simulink model "SAR_ADC_Resistive_DAC_SinInput_HighSpeed_12072024"  (R2022a)
settings: Solver=VariableStepAuto  StartTime=0.0  StopTime=5e-5  RelTol=1e-3
libraries: fl_lib x93, nesl_utility x28, simulink_extras x11, ee_lib x10
settings Model: Creator=subha  LastModifiedBy=subha

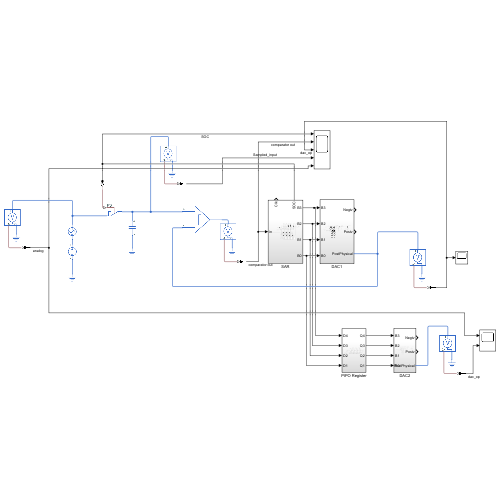
[thumbnail: Simulink's stored preview of the top-level diagram]
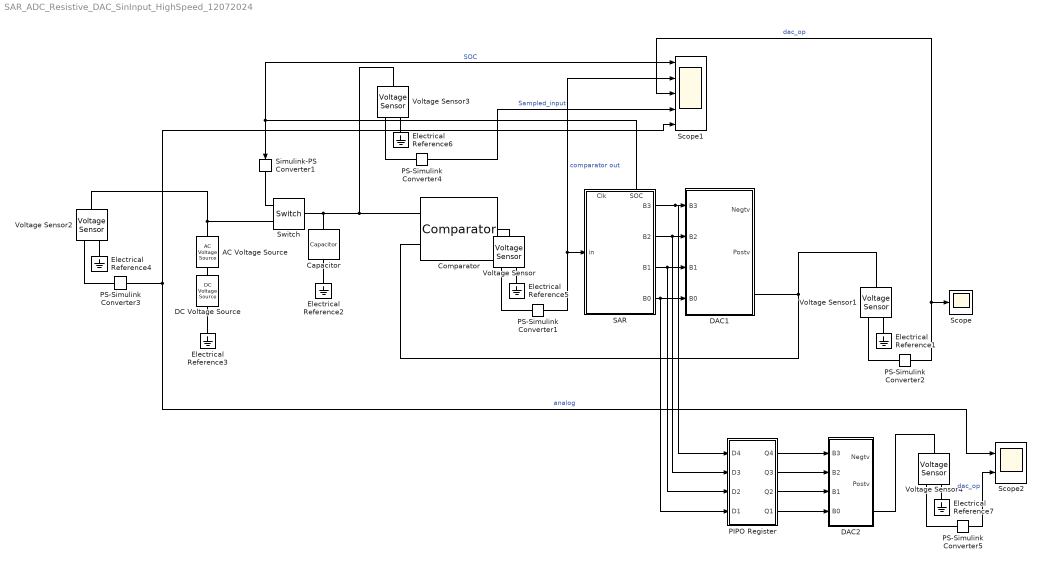
== system SAR_ADC_Resistive_DAC_SinInput_HighSpeed_12072024 ==
  AC Voltage Source : fl_lib/Electrical/Electrical Sources/AC Voltage Source  amp=0.9 V  shift=0 deg  frequency=0.1 MHz  omega=0 rad/s
      settings: SourceProductBaseCode=PW,SS,VE
  Capacitor : fl_lib/Electrical/Electrical Elements/Capacitor  c=1e-9 F  r=1e-6 Ohm  g=0 1/Ohm  i_specify=off  i_priority=None  i=0 A  i_nominal_specify=off  i_nominal_unit=A  i_nominal_value=1  v_specify=off  v_priority=None  v=0 V  v_nominal_specify=off  v_nominal_unit=V  v_nominal_value=1  vc_specify=off  vc_priority=High  vc=0 V  vc_nominal_specify=off  vc_nominal_unit=V  vc_nominal_value=1
      settings: SourceProductBaseCode=PW,SS,VE
  Comparator : ee_lib/Integrated Circuits/Comparator  V_OS=5 mV  C_IN=0 pF  V_OL=0 V  V_OH=5 V  R_OUT=50 Ohm  Delay=0 s
      settings: SourceProductBaseCode=PS  InternalSimscapePortConfiguration="{\"Bottom\":[],\"Left\":[{\"id\":\"p\",\"label\":\"+\",\"type\":\"foundation.electrical.electrical\"},{\"id\":\"n\",\"label\":\"-\",\"type\":\"foundation.electrical.electrical\"}],\"Right\":[{\"id\":\"J\",\"label\":\"\",\"type\":\"foundation.electrical.electrical\"}],\"Top\":[]}"
  DAC1 : Subsystem
  DAC2 : Subsystem
  DC Voltage Source : ee_lib/Additional Components/SPICE Sources/DC Voltage Source  DC=0.9 V
  Electrical Reference{1..7} (7 alike) : fl_lib/Electrical/Electrical Elements/Electrical Reference
      settings: SourceProductBaseCode=PW,SS,VE
  PIPO Register : Subsystem
  PS-Simulink Converter{1..5} (5 alike) : nesl_utility/PS-Simulink Converter  PhysicalDomain=network_engine_domain  SubClassName=ps_output  LeftPortType=input  RightPortType=output  PseudoPeriodic=off  Frequencies=[]  VectorFormat=inherit  Unit=inherit  AffineConversion=off
      settings: SourceProductBaseCode=SS,PW,VE
  SAR : Subsystem
      settings: PortSchema="{\"entries\":[{\"content\":{\"sides\":[{\"content\":{\"connectorIds\":[\"In1\"]},\"type\":\"ConnectorPlacement.EquallySpacedRectSide\",\"uuid\":\"d83d6cbf-1b3c-43c1-b494-336f4d7c2172\"},{\"content\":{\"connectorIds\":[\"Out1\",\"Out2\",\"Out3\",\"Out4\"],\"side\":\"RIGHT\"},\"type\":\"ConnectorPlacement.EquallySpacedRectSide\",\"uuid\":\"5d3d46d0-2210-4ca5-910c-914e08ba7e35\"},{\"content\":{\"connectorIds\":[\"Out5\",\"Out6\"],\"side\":\"TOP\"},\"type\":\"ConnectorPlacement.EquallySpacedRectSide\",\"uuid\":\"cdad274f-a51a-4eb7-9d94-8deabecbb179\"}]},\"type\":\"ConnectorPlacement.EquallySpacedConnector\",\"uuid\":\"7d06527c-7ef1-4315-9939-5225cbeec2df\"}],\"packageUris\":[\"http://schema.mathworks.com/mf0/Connector/R2020b\"],\"version\":\"1.0\"}"
  Scope : Scope
  Scope1 : Scope  NumInputPorts=5
  Scope2 : Scope  NumInputPorts=2
  Simulink-PS Converter1 : nesl_utility/Simulink-PS Converter  PhysicalDomain=network_engine_domain  SubClassName=ps_input  LeftPortType=input  RightPortType=output  PseudoPeriodic=off  Frequencies=[]  NoiseDistribution=none  NoiseParameters=[]  Unit=1  AffineConversion=off  FilteringAndDerivatives=provide  SimscapeFilterOrder=1  InputFilterTimeConstant=0.001  UdotUserProvided=0
      settings: SourceProductBaseCode=SS,PW,VE
  Switch : fl_lib/Electrical/Electrical Elements/Switch  R_closed=0.01 Ohm  G_open=1e-10 1/Ohm  Threshold=0.5  i_specify=off  i_priority=None  i=0 A  i_nominal_specify=off  i_nominal_unit=A  i_nominal_value=1  v_specify=off  v_priority=None  v=0 V  v_nominal_specify=off  v_nominal_unit=V  v_nominal_value=1
      settings: SourceProductBaseCode=PW,SS,VE
  Voltage Sensor{,1..4} (5 alike) : fl_lib/Electrical/Electrical Sensors/Voltage Sensor
      settings: SourceProductBaseCode=PW,SS,VE
  wires:
  PS-Simulink Converter2/1 -> Scope1/3, Scope/1  "dac_op"
  SAR/4(B0) -> DAC1/4(B0), PIPO Register/4(D1)
  PS-Simulink Converter4/1 -> Scope1/4  "Sampled_input"
  PS-Simulink Converter1/1 -> Scope1/2, SAR/1(in)  "comparator out"
  SAR/3(B1) -> PIPO Register/3(D2), DAC1/3(B1)
  SAR/1(B3) -> PIPO Register/1(D4), DAC1/1(B3)
  SAR/2(B2) -> PIPO Register/2(D3), DAC1/2(B2)
  SAR/6(SOC) -> Simulink-PS Converter1/1, Scope1/1  "SOC"
  PS-Simulink Converter3/1 -> Scope2/1, Scope1/5  "analog"
  PIPO Register/1(Q4) -> DAC2/1(B3)
  PIPO Register/2(Q3) -> DAC2/2(B2)
  PIPO Register/3(Q2) -> DAC2/3(B1)
  PIPO Register/4(Q1) -> DAC2/4(B0)
  PS-Simulink Converter5/1 -> Scope2/2  "dac_op"
  connections:
  Capacitor/LConn1 -- Switch/LConn1 -- Comparator/LConn1 -- Voltage Sensor3/LConn1
  Comparator/LConn2 -- DAC1/RConn1 -- Voltage Sensor1/LConn1
  Electrical Reference6/LConn1 -- Voltage Sensor3/RConn2
  Voltage Sensor1/RConn1 -- PS-Simulink Converter2/LConn1
  Simulink-PS Converter1/RConn1 -- Switch/RConn1
  Voltage Sensor3/RConn1 -- PS-Simulink Converter4/LConn1
  Electrical Reference2/LConn1 -- Capacitor/RConn1
  Electrical Reference5/LConn1 -- Voltage Sensor/RConn2
  Voltage Sensor/RConn1 -- PS-Simulink Converter1/LConn1
  Comparator/RConn1 -- Voltage Sensor/LConn1
  Electrical Reference1/LConn1 -- Voltage Sensor1/RConn2
  AC Voltage Source/LConn1 -- Voltage Sensor2/LConn1 -- Switch/RConn2
  DC Voltage Source/LConn1 -- AC Voltage Source/RConn1
  DC Voltage Source/RConn1 -- Electrical Reference3/LConn1
  Electrical Reference4/LConn1 -- Voltage Sensor2/RConn2
  Voltage Sensor2/RConn1 -- PS-Simulink Converter3/LConn1
  Voltage Sensor4/RConn1 -- PS-Simulink Converter5/LConn1
  Electrical Reference7/LConn1 -- Voltage Sensor4/RConn2
  DAC2/RConn1 -- Voltage Sensor4/LConn1

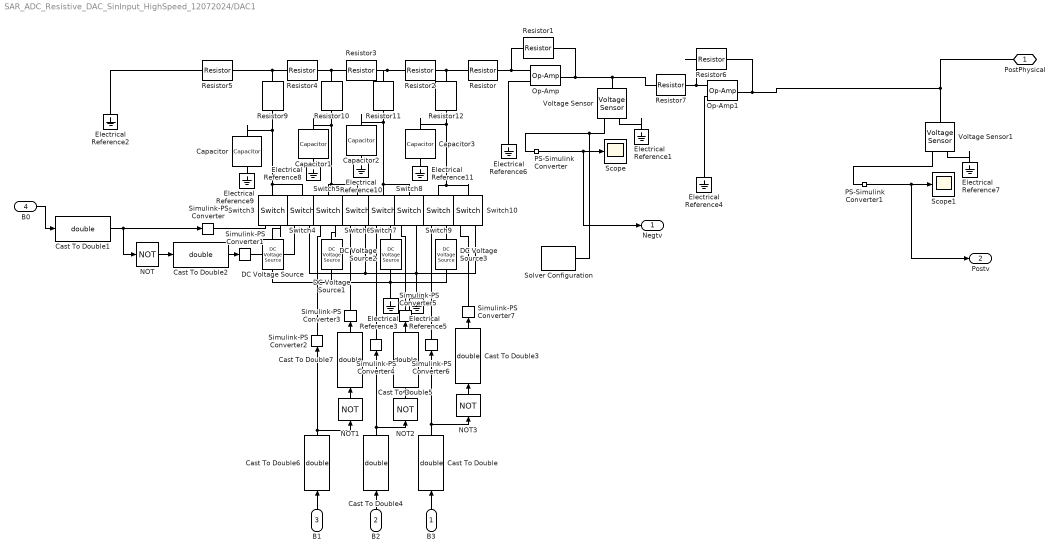
== system SAR_ADC_Resistive_DAC_SinInput_HighSpeed_12072024/DAC1 ==
  B3 : Inport
  B2 : Inport  Port=2
  B1 : Inport  Port=3
  B0 : Inport  Port=4
  Capacitor{,1..3} (4 alike) : fl_lib/Electrical/Electrical Elements/Capacitor  c=1e-9 F  r=1e-6 Ohm  g=0 1/Ohm  i_specify=off  i_priority=None  i=0 A  i_nominal_specify=off  i_nominal_unit=A  i_nominal_value=1  v_specify=off  v_priority=None  v=0 V  v_nominal_specify=off  v_nominal_unit=V  v_nominal_value=1  vc_specify=off  vc_priority=High  vc=0 V  vc_nominal_specify=off  vc_nominal_unit=V  vc_nominal_value=1
      settings: SourceProductBaseCode=PW,SS,VE
  Cast To Double{,1..7} (8 alike) : DataTypeConversion  OutDataTypeStr=double  SaturateOnIntegerOverflow=off  RndMeth=Floor
  DC Voltage Source{,1..3} (4 alike) : ee_lib/Additional Components/SPICE Sources/DC Voltage Source  DC=1.8 V
  Electrical Reference{1..11} (11 alike) : fl_lib/Electrical/Electrical Elements/Electrical Reference
      settings: SourceProductBaseCode=PW,SS,VE
  NOT{,1..3} (4 alike) : Logic  Operator=NOT  IconShape=distinctive  AllPortsSameDT=off  OutDataTypeStr=boolean
  Op-Amp : fl_lib/Electrical/Electrical Elements/Op-Amp  outI_specify=off  outI_priority=None  outI=0 A  outI_nominal_specify=off  outI_nominal_unit=A  outI_nominal_value=1
      settings: SourceProductBaseCode=PW,SS,VE
  Op-Amp1 : fl_lib/Electrical/Electrical Elements/Op-Amp  outI_specify=off  outI_priority=None  outI=0 A  outI_nominal_specify=off  outI_nominal_unit=A  outI_nominal_value=1
      settings: SourceProductBaseCode=PW,SS,VE
  PS-Simulink Converter : nesl_utility/PS-Simulink Converter  PhysicalDomain=network_engine_domain  SubClassName=ps_output  LeftPortType=input  RightPortType=output  PseudoPeriodic=off  Frequencies=[]  VectorFormat=inherit  Unit=inherit  AffineConversion=off
      settings: SourceProductBaseCode=SS,PW,VE
  PS-Simulink Converter1 : nesl_utility/PS-Simulink Converter  PhysicalDomain=network_engine_domain  SubClassName=ps_output  LeftPortType=input  RightPortType=output  PseudoPeriodic=off  Frequencies=[]  VectorFormat=inherit  Unit=inherit  AffineConversion=off
      settings: SourceProductBaseCode=SS,PW,VE
  Resistor{,2..4} (4 alike) : fl_lib/Electrical/Electrical Elements/Resistor  R=1 kOhm  i_specify=off  i_priority=None  i=0 A  i_nominal_specify=off  i_nominal_unit=A  i_nominal_value=1  v_specify=off  v_priority=None  v=0 V  v_nominal_specify=off  v_nominal_unit=V  v_nominal_value=1
      settings: SourceProductBaseCode=PW,SS,VE
  Resistor{1,5,9..12} (6 alike) : fl_lib/Electrical/Electrical Elements/Resistor  R=2 kOhm  i_specify=off  i_priority=None  i=0 A  i_nominal_specify=off  i_nominal_unit=A  i_nominal_value=1  v_specify=off  v_priority=None  v=0 V  v_nominal_specify=off  v_nominal_unit=V  v_nominal_value=1
      settings: SourceProductBaseCode=PW,SS,VE
  Resistor6 : fl_lib/Electrical/Electrical Elements/Resistor  R=10 kOhm  i_specify=off  i_priority=None  i=0 A  i_nominal_specify=off  i_nominal_unit=A  i_nominal_value=1  v_specify=off  v_priority=None  v=0 V  v_nominal_specify=off  v_nominal_unit=V  v_nominal_value=1
      settings: SourceProductBaseCode=PW,SS,VE
  Resistor7 : fl_lib/Electrical/Electrical Elements/Resistor  R=10 kOhm  i_specify=off  i_priority=None  i=0 A  i_nominal_specify=off  i_nominal_unit=A  i_nominal_value=1  v_specify=off  v_priority=None  v=0 V  v_nominal_specify=off  v_nominal_unit=V  v_nominal_value=1
      settings: SourceProductBaseCode=PW,SS,VE
  Scope : Scope
  Scope1 : Scope
  Simulink-PS Converter{,1..7} (8 alike) : nesl_utility/Simulink-PS Converter  PhysicalDomain=network_engine_domain  SubClassName=ps_input  LeftPortType=input  RightPortType=output  PseudoPeriodic=off  Frequencies=[]  NoiseDistribution=none  NoiseParameters=[]  Unit=1  AffineConversion=off  FilteringAndDerivatives=provide  SimscapeFilterOrder=1  InputFilterTimeConstant=0.001  UdotUserProvided=0
      settings: SourceProductBaseCode=SS,PW,VE
  Solver Configuration : nesl_utility/Solver Configuration  PhysicalDomain=network_engine_domain  SubClassName=solver  LeftPortType=input  RightPortType=generic  Tones=[]  Harmonics=[]  SimulateNoise=off  Profile=off  UseLocalSampling=off  EnableSwitchedLinearOptims=on  FrequencyDomain=off  UseCCode=off  RelTol=0.001  AbsTol=0.001  MinStep=1e-09  ToWorkspace=off  RevertToSquareIcSolve=off  NumHomotopyIterations=100  PhasorMode=off  PhasorModeNumHarmonics=1  IndexReductionMethod=DerivativeReplacement  DoDC=off  ResidualTolerance=1e-09  UseLocalSolver=off  LocalSolverChoice=NE_BACKWARD_EULER_ADVANCER  LocalSolverSampleTime=0.001  DoFixedCost=off  MaxNonlinIter=3  MaxModeIter=2  ComputeImpulses=off  ImpulseIterations=2  LinearAlgebra=auto  LinearAlgebraNumThread=0  EquationFormulation=NE_TIME_EF  DelaysMemoryBudget=1024  AutomaticFiltering=on  FilteringTimeConstant=0.001  PartitionStorageMethod=AS_NEEDED  PartitionMemoryBudget=1024  PartitionMethod=ROBUST
      settings: SourceProductBaseCode=SS,PW,VE
  Switch{3..10} (8 alike) : fl_lib/Electrical/Electrical Elements/Switch  R_closed=0.01 Ohm  G_open=1e-8 1/Ohm  Threshold=0.5  i_specify=off  i_priority=None  i=0 A  i_nominal_specify=off  i_nominal_unit=A  i_nominal_value=1  v_specify=off  v_priority=None  v=0 V  v_nominal_specify=off  v_nominal_unit=V  v_nominal_value=1
      settings: SourceProductBaseCode=PW,SS,VE
  Voltage Sensor : fl_lib/Electrical/Electrical Sensors/Voltage Sensor
      settings: SourceProductBaseCode=PW,SS,VE
  Voltage Sensor1 : fl_lib/Electrical/Electrical Sensors/Voltage Sensor
      settings: SourceProductBaseCode=PW,SS,VE
  PostPhysical : PMIOPort  Side=Right
  Negtv : Outport
  Postv : Outport  Port=2
  wires:
  PS-Simulink Converter/1 -> Negtv/1, Scope/1
  Cast To Double/1 -> Simulink-PS Converter6/1, NOT3/1
  B3/1 -> Cast To Double/1
  B0/1 -> Cast To Double1/1
  Cast To Double1/1 -> Simulink-PS Converter/1, NOT/1
  NOT/1 -> Cast To Double2/1
  Cast To Double2/1 -> Simulink-PS Converter1/1
  Cast To Double3/1 -> Simulink-PS Converter7/1
  NOT3/1 -> Cast To Double3/1
  B2/1 -> Cast To Double4/1
  Cast To Double4/1 -> NOT2/1, Simulink-PS Converter4/1
  NOT2/1 -> Cast To Double5/1
  Cast To Double5/1 -> Simulink-PS Converter5/1
  B1/1 -> Cast To Double6/1
  Cast To Double6/1 -> NOT1/1, Simulink-PS Converter2/1
  NOT1/1 -> Cast To Double7/1
  Cast To Double7/1 -> Simulink-PS Converter3/1
  PS-Simulink Converter1/1 -> Postv/1, Scope1/1
  connections:
  Voltage Sensor/RConn1 -- Solver Configuration/RConn1 -- PS-Simulink Converter/LConn1
  DC Voltage Source/RConn1 -- DC Voltage Source1/RConn1 -- DC Voltage Source2/RConn1 -- Electrical Reference3/LConn1 -- DC Voltage Source3/RConn1
  Resistor3/RConn1 -- Resistor2/LConn1 -- Resistor11/LConn1
  Resistor4/RConn1 -- Resistor10/LConn1 -- Resistor3/LConn1
  Resistor5/RConn1 -- Resistor4/LConn1 -- Resistor9/LConn1
  Electrical Reference1/LConn1 -- Voltage Sensor/RConn2
  Resistor2/RConn1 -- Resistor/LConn1 -- Resistor12/LConn1
  Op-Amp/RConn1 -- Resistor7/LConn1 -- Voltage Sensor/LConn1 -- Resistor1/RConn1
  Resistor/RConn1 -- Resistor1/LConn1 -- Op-Amp/LConn2
  Electrical Reference6/LConn1 -- Op-Amp/LConn1
  Switch3/LConn1 -- Switch4/LConn1 -- Capacitor/LConn1 -- Resistor9/RConn1
  Switch3/RConn2 -- DC Voltage Source/LConn1
  Electrical Reference5/LConn1 -- Switch10/RConn2 -- Switch4/RConn2 -- Switch6/RConn2 -- Switch8/RConn2
  Simulink-PS Converter1/RConn1 -- Switch4/RConn1
  Switch5/LConn1 -- Switch6/LConn1 -- Capacitor1/LConn1 -- Resistor10/RConn1
  Switch5/RConn2 -- DC Voltage Source1/LConn1
  Switch7/LConn1 -- Switch8/LConn1 -- Capacitor2/LConn1 -- Resistor11/RConn1
  Switch7/RConn2 -- DC Voltage Source2/LConn1
  Switch10/LConn1 -- Capacitor3/LConn1 -- Resistor12/RConn1 -- Switch9/LConn1
  Switch9/RConn2 -- DC Voltage Source3/LConn1
  Simulink-PS Converter/RConn1 -- Switch3/RConn1
  Simulink-PS Converter3/RConn1 -- Switch6/RConn1
  Simulink-PS Converter2/RConn1 -- Switch5/RConn1
  Switch7/RConn1 -- Simulink-PS Converter4/RConn1
  Switch8/RConn1 -- Simulink-PS Converter5/RConn1
  Switch9/RConn1 -- Simulink-PS Converter6/RConn1
  Switch10/RConn1 -- Simulink-PS Converter7/RConn1
  Electrical Reference4/LConn1 -- Op-Amp1/LConn1
  Resistor7/RConn1 -- Op-Amp1/LConn2 -- Resistor6/LConn1
  Voltage Sensor1/RConn1 -- PS-Simulink Converter1/LConn1
  Resistor6/RConn1 -- Op-Amp1/RConn1 -- PostPhysical/RConn1 -- Voltage Sensor1/LConn1
  Electrical Reference7/LConn1 -- Voltage Sensor1/RConn2
  Electrical Reference2/LConn1 -- Resistor5/LConn1
  Electrical Reference9/LConn1 -- Capacitor/RConn1
  Electrical Reference8/LConn1 -- Capacitor1/RConn1
  Electrical Reference10/LConn1 -- Capacitor2/RConn1
  Electrical Reference11/LConn1 -- Capacitor3/RConn1

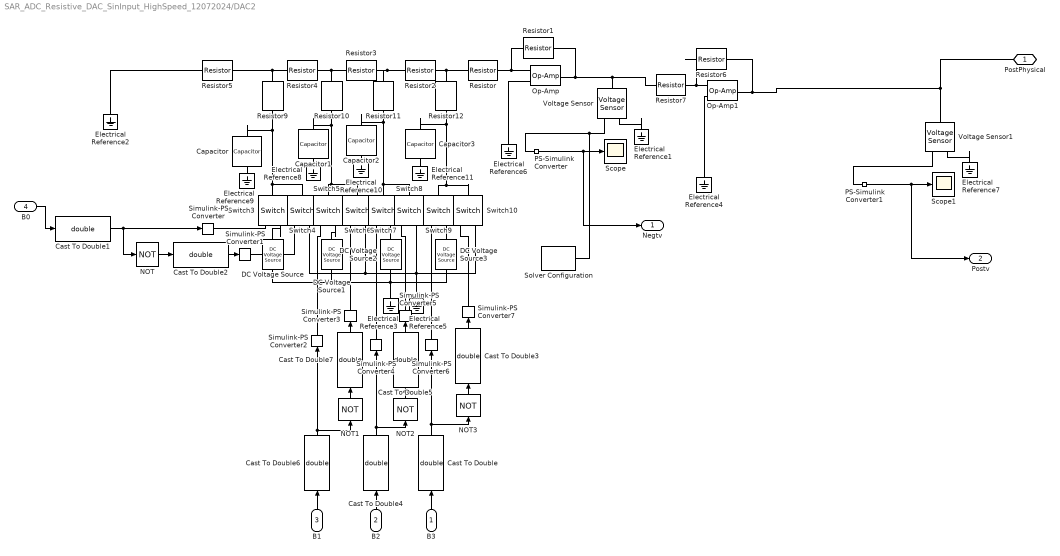
== system SAR_ADC_Resistive_DAC_SinInput_HighSpeed_12072024/DAC2 ==
  B3 : Inport
  B2 : Inport  Port=2
  B1 : Inport  Port=3
  B0 : Inport  Port=4
  Capacitor{,1..3} (4 alike) : fl_lib/Electrical/Electrical Elements/Capacitor  c=1e-9 F  r=1e-6 Ohm  g=0 1/Ohm  i_specify=off  i_priority=None  i=0 A  i_nominal_specify=off  i_nominal_unit=A  i_nominal_value=1  v_specify=off  v_priority=None  v=0 V  v_nominal_specify=off  v_nominal_unit=V  v_nominal_value=1  vc_specify=off  vc_priority=High  vc=0 V  vc_nominal_specify=off  vc_nominal_unit=V  vc_nominal_value=1
      settings: SourceProductBaseCode=PW,SS,VE
  Cast To Double{,1..7} (8 alike) : DataTypeConversion  OutDataTypeStr=double  SaturateOnIntegerOverflow=off  RndMeth=Floor
  DC Voltage Source{,1..3} (4 alike) : ee_lib/Additional Components/SPICE Sources/DC Voltage Source  DC=1.8 V
  Electrical Reference{1..11} (11 alike) : fl_lib/Electrical/Electrical Elements/Electrical Reference
      settings: SourceProductBaseCode=PW,SS,VE
  NOT{,1..3} (4 alike) : Logic  Operator=NOT  IconShape=distinctive  AllPortsSameDT=off  OutDataTypeStr=boolean
  Op-Amp : fl_lib/Electrical/Electrical Elements/Op-Amp  outI_specify=off  outI_priority=None  outI=0 A  outI_nominal_specify=off  outI_nominal_unit=A  outI_nominal_value=1
      settings: SourceProductBaseCode=PW,SS,VE
  Op-Amp1 : fl_lib/Electrical/Electrical Elements/Op-Amp  outI_specify=off  outI_priority=None  outI=0 A  outI_nominal_specify=off  outI_nominal_unit=A  outI_nominal_value=1
      settings: SourceProductBaseCode=PW,SS,VE
  PS-Simulink Converter : nesl_utility/PS-Simulink Converter  PhysicalDomain=network_engine_domain  SubClassName=ps_output  LeftPortType=input  RightPortType=output  PseudoPeriodic=off  Frequencies=[]  VectorFormat=inherit  Unit=inherit  AffineConversion=off
      settings: SourceProductBaseCode=SS,PW,VE
  PS-Simulink Converter1 : nesl_utility/PS-Simulink Converter  PhysicalDomain=network_engine_domain  SubClassName=ps_output  LeftPortType=input  RightPortType=output  PseudoPeriodic=off  Frequencies=[]  VectorFormat=inherit  Unit=inherit  AffineConversion=off
      settings: SourceProductBaseCode=SS,PW,VE
  Resistor{,2..4} (4 alike) : fl_lib/Electrical/Electrical Elements/Resistor  R=1 kOhm  i_specify=off  i_priority=None  i=0 A  i_nominal_specify=off  i_nominal_unit=A  i_nominal_value=1  v_specify=off  v_priority=None  v=0 V  v_nominal_specify=off  v_nominal_unit=V  v_nominal_value=1
      settings: SourceProductBaseCode=PW,SS,VE
  Resistor{1,5,9..12} (6 alike) : fl_lib/Electrical/Electrical Elements/Resistor  R=2 kOhm  i_specify=off  i_priority=None  i=0 A  i_nominal_specify=off  i_nominal_unit=A  i_nominal_value=1  v_specify=off  v_priority=None  v=0 V  v_nominal_specify=off  v_nominal_unit=V  v_nominal_value=1
      settings: SourceProductBaseCode=PW,SS,VE
  Resistor6 : fl_lib/Electrical/Electrical Elements/Resistor  R=10 kOhm  i_specify=off  i_priority=None  i=0 A  i_nominal_specify=off  i_nominal_unit=A  i_nominal_value=1  v_specify=off  v_priority=None  v=0 V  v_nominal_specify=off  v_nominal_unit=V  v_nominal_value=1
      settings: SourceProductBaseCode=PW,SS,VE
  Resistor7 : fl_lib/Electrical/Electrical Elements/Resistor  R=10 kOhm  i_specify=off  i_priority=None  i=0 A  i_nominal_specify=off  i_nominal_unit=A  i_nominal_value=1  v_specify=off  v_priority=None  v=0 V  v_nominal_specify=off  v_nominal_unit=V  v_nominal_value=1
      settings: SourceProductBaseCode=PW,SS,VE
  Scope : Scope
  Scope1 : Scope
  Simulink-PS Converter{,1..7} (8 alike) : nesl_utility/Simulink-PS Converter  PhysicalDomain=network_engine_domain  SubClassName=ps_input  LeftPortType=input  RightPortType=output  PseudoPeriodic=off  Frequencies=[]  NoiseDistribution=none  NoiseParameters=[]  Unit=1  AffineConversion=off  FilteringAndDerivatives=provide  SimscapeFilterOrder=1  InputFilterTimeConstant=0.001  UdotUserProvided=0
      settings: SourceProductBaseCode=SS,PW,VE
  Solver Configuration : nesl_utility/Solver Configuration  PhysicalDomain=network_engine_domain  SubClassName=solver  LeftPortType=input  RightPortType=generic  Tones=[]  Harmonics=[]  SimulateNoise=off  Profile=off  UseLocalSampling=off  EnableSwitchedLinearOptims=on  FrequencyDomain=off  UseCCode=off  RelTol=0.001  AbsTol=0.001  MinStep=1e-09  ToWorkspace=off  RevertToSquareIcSolve=off  NumHomotopyIterations=100  PhasorMode=off  PhasorModeNumHarmonics=1  IndexReductionMethod=DerivativeReplacement  DoDC=off  ResidualTolerance=1e-09  UseLocalSolver=off  LocalSolverChoice=NE_BACKWARD_EULER_ADVANCER  LocalSolverSampleTime=0.001  DoFixedCost=off  MaxNonlinIter=3  MaxModeIter=2  ComputeImpulses=off  ImpulseIterations=2  LinearAlgebra=auto  LinearAlgebraNumThread=0  EquationFormulation=NE_TIME_EF  DelaysMemoryBudget=1024  AutomaticFiltering=on  FilteringTimeConstant=0.001  PartitionStorageMethod=AS_NEEDED  PartitionMemoryBudget=1024  PartitionMethod=ROBUST
      settings: SourceProductBaseCode=SS,PW,VE
  Switch{3..10} (8 alike) : fl_lib/Electrical/Electrical Elements/Switch  R_closed=0.01 Ohm  G_open=1e-8 1/Ohm  Threshold=0.5  i_specify=off  i_priority=None  i=0 A  i_nominal_specify=off  i_nominal_unit=A  i_nominal_value=1  v_specify=off  v_priority=None  v=0 V  v_nominal_specify=off  v_nominal_unit=V  v_nominal_value=1
      settings: SourceProductBaseCode=PW,SS,VE
  Voltage Sensor : fl_lib/Electrical/Electrical Sensors/Voltage Sensor
      settings: SourceProductBaseCode=PW,SS,VE
  Voltage Sensor1 : fl_lib/Electrical/Electrical Sensors/Voltage Sensor
      settings: SourceProductBaseCode=PW,SS,VE
  PostPhysical : PMIOPort  Side=Right
  Negtv : Outport
  Postv : Outport  Port=2
  wires:
  PS-Simulink Converter/1 -> Negtv/1, Scope/1
  Cast To Double/1 -> Simulink-PS Converter6/1, NOT3/1
  B3/1 -> Cast To Double/1
  B0/1 -> Cast To Double1/1
  Cast To Double1/1 -> Simulink-PS Converter/1, NOT/1
  NOT/1 -> Cast To Double2/1
  Cast To Double2/1 -> Simulink-PS Converter1/1
  Cast To Double3/1 -> Simulink-PS Converter7/1
  NOT3/1 -> Cast To Double3/1
  B2/1 -> Cast To Double4/1
  Cast To Double4/1 -> NOT2/1, Simulink-PS Converter4/1
  NOT2/1 -> Cast To Double5/1
  Cast To Double5/1 -> Simulink-PS Converter5/1
  B1/1 -> Cast To Double6/1
  Cast To Double6/1 -> NOT1/1, Simulink-PS Converter2/1
  NOT1/1 -> Cast To Double7/1
  Cast To Double7/1 -> Simulink-PS Converter3/1
  PS-Simulink Converter1/1 -> Postv/1, Scope1/1
  connections:
  Voltage Sensor/RConn1 -- Solver Configuration/RConn1 -- PS-Simulink Converter/LConn1
  DC Voltage Source/RConn1 -- DC Voltage Source1/RConn1 -- DC Voltage Source2/RConn1 -- Electrical Reference3/LConn1 -- DC Voltage Source3/RConn1
  Resistor3/RConn1 -- Resistor2/LConn1 -- Resistor11/LConn1
  Resistor4/RConn1 -- Resistor10/LConn1 -- Resistor3/LConn1
  Resistor5/RConn1 -- Resistor4/LConn1 -- Resistor9/LConn1
  Electrical Reference1/LConn1 -- Voltage Sensor/RConn2
  Resistor2/RConn1 -- Resistor/LConn1 -- Resistor12/LConn1
  Op-Amp/RConn1 -- Resistor7/LConn1 -- Voltage Sensor/LConn1 -- Resistor1/RConn1
  Resistor/RConn1 -- Resistor1/LConn1 -- Op-Amp/LConn2
  Electrical Reference6/LConn1 -- Op-Amp/LConn1
  Switch3/LConn1 -- Switch4/LConn1 -- Capacitor/LConn1 -- Resistor9/RConn1
  Switch3/RConn2 -- DC Voltage Source/LConn1
  Electrical Reference5/LConn1 -- Switch10/RConn2 -- Switch4/RConn2 -- Switch6/RConn2 -- Switch8/RConn2
  Simulink-PS Converter1/RConn1 -- Switch4/RConn1
  Switch5/LConn1 -- Switch6/LConn1 -- Capacitor1/LConn1 -- Resistor10/RConn1
  Switch5/RConn2 -- DC Voltage Source1/LConn1
  Switch7/LConn1 -- Switch8/LConn1 -- Capacitor2/LConn1 -- Resistor11/RConn1
  Switch7/RConn2 -- DC Voltage Source2/LConn1
  Switch10/LConn1 -- Capacitor3/LConn1 -- Resistor12/RConn1 -- Switch9/LConn1
  Switch9/RConn2 -- DC Voltage Source3/LConn1
  Simulink-PS Converter/RConn1 -- Switch3/RConn1
  Simulink-PS Converter3/RConn1 -- Switch6/RConn1
  Simulink-PS Converter2/RConn1 -- Switch5/RConn1
  Switch7/RConn1 -- Simulink-PS Converter4/RConn1
  Switch8/RConn1 -- Simulink-PS Converter5/RConn1
  Switch9/RConn1 -- Simulink-PS Converter6/RConn1
  Switch10/RConn1 -- Simulink-PS Converter7/RConn1
  Electrical Reference4/LConn1 -- Op-Amp1/LConn1
  Resistor7/RConn1 -- Op-Amp1/LConn2 -- Resistor6/LConn1
  Voltage Sensor1/RConn1 -- PS-Simulink Converter1/LConn1
  Resistor6/RConn1 -- Op-Amp1/RConn1 -- PostPhysical/RConn1 -- Voltage Sensor1/LConn1
  Electrical Reference7/LConn1 -- Voltage Sensor1/RConn2
  Electrical Reference2/LConn1 -- Resistor5/LConn1
  Electrical Reference9/LConn1 -- Capacitor/RConn1
  Electrical Reference8/LConn1 -- Capacitor1/RConn1
  Electrical Reference10/LConn1 -- Capacitor2/RConn1
  Electrical Reference11/LConn1 -- Capacitor3/RConn1

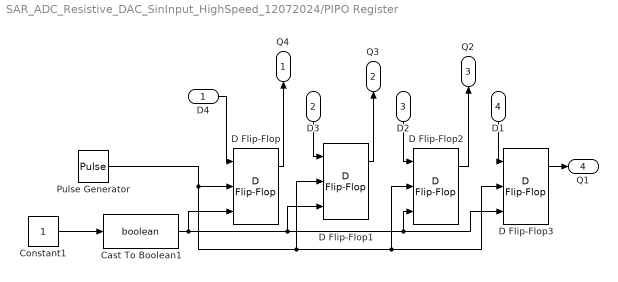
== system SAR_ADC_Resistive_DAC_SinInput_HighSpeed_12072024/PIPO Register ==
  D4 : Inport
  D3 : Inport  Port=2
  D2 : Inport  Port=3
  D1 : Inport  Port=4
  Cast To Boolean1 : DataTypeConversion  OutDataTypeStr=boolean  SaturateOnIntegerOverflow=off  RndMeth=Floor
  Constant1 : Constant
  D Flip-Flop{,1..3} (4 alike) : simulink_extras/Flip Flops/D Flip-Flop
  Pulse Generator : DiscretePulseGenerator  PulseType=Time based  Period=12e-8  PulseWidth=8.3  PhaseDelay=11e-8
  Q4 : Outport
  Q3 : Outport  Port=2
  Q2 : Outport  Port=3
  Q1 : Outport  Port=4
  wires:
  Constant1/1 -> Cast To Boolean1/1
  Pulse Generator/1 -> D Flip-Flop3/2, D Flip-Flop2/2, D Flip-Flop1/2, D Flip-Flop/2
  D1/1 -> D Flip-Flop3/1
  Cast To Boolean1/1 -> D Flip-Flop2/3, D Flip-Flop3/3, D Flip-Flop1/3, D Flip-Flop/3
  D Flip-Flop/1 -> Q4/1
  D Flip-Flop2/1 -> Q2/1
  D2/1 -> D Flip-Flop2/1
  D3/1 -> D Flip-Flop1/1
  D Flip-Flop3/1 -> Q1/1
  D Flip-Flop1/1 -> Q3/1
  D4/1 -> D Flip-Flop/1

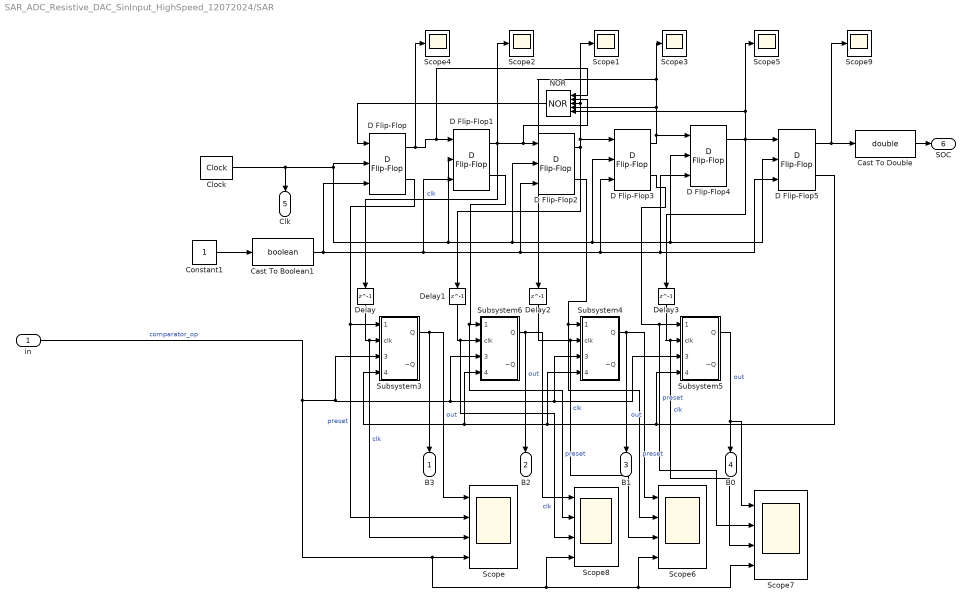
== system SAR_ADC_Resistive_DAC_SinInput_HighSpeed_12072024/SAR ==
  in : Inport
  Cast To Boolean1 : DataTypeConversion  OutDataTypeStr=boolean  SaturateOnIntegerOverflow=off  RndMeth=Floor
  Cast To Double : DataTypeConversion  OutDataTypeStr=double  SaturateOnIntegerOverflow=off  RndMeth=Floor
  Clock : simulink_extras/Flip Flops/Clock  period=2e-8
  Constant1 : Constant
  D Flip-Flop{,1..5} (6 alike) : simulink_extras/Flip Flops/D Flip-Flop
  Delay{,1..3} (4 alike) : Delay  DelayLength=1
  NOR : Logic  Operator=NOR  Inputs=5  IconShape=distinctive  AllPortsSameDT=off  OutDataTypeStr=boolean
  Scope{,6..8} (4 alike) : Scope  NumInputPorts=4
  Scope{1..5,9} (6 alike) : Scope
  Subsystem3 : Subsystem
  Subsystem4 : Subsystem
  Subsystem5 : Subsystem
  Subsystem6 : Subsystem
  B3 : Outport
  B2 : Outport  Port=2
  B1 : Outport  Port=3
  B0 : Outport  Port=4
  Clk : Outport  Port=5
  SOC : Outport  Port=6
  wires:
  D Flip-Flop3/1 -> NOR/4, Delay2/1, Scope3/1, D Flip-Flop4/1
  Clock/1 -> Clk/1, D Flip-Flop/2, D Flip-Flop1/2, D Flip-Flop2/2, D Flip-Flop5/2, D Flip-Flop4/2, D Flip-Flop3/2
  D Flip-Flop3/2 -> Scope7/2, Subsystem5/1(preset)  "preset"
  in/1 -> Scope7/4, Scope6/4, Scope8/4, Scope/4, Subsystem3/3(input), Subsystem6/3(input), Subsystem5/3(input), Subsystem4/3(input)  "comparator_op"
  NOR/1 -> D Flip-Flop/1
  Delay2/1 -> Scope6/3, Subsystem4/2(clk)  "clk"
  Delay3/1 -> Scope7/3, Subsystem5/2(clk)  "clk"
  D Flip-Flop4/1 -> D Flip-Flop5/1, Delay3/1, NOR/5, Scope5/1
  Cast To Boolean1/1 -> D Flip-Flop/3, D Flip-Flop5/3, D Flip-Flop4/3, D Flip-Flop3/3, D Flip-Flop2/3, D Flip-Flop1/3
  D Flip-Flop2/2 -> Scope6/2, Subsystem4/1(preset)  "preset"
  D Flip-Flop1/2 -> Scope8/2, Subsystem6/1(preset)  "preset"
  D Flip-Flop2/1 -> Delay1/1, D Flip-Flop3/1, NOR/3, Scope1/1
  D Flip-Flop1/1 -> Delay/1, NOR/2, D Flip-Flop2/1, Scope2/1  "clk"
  Subsystem6/1(Q) -> B2/1, Scope8/1  "out"
  D Flip-Flop/1 -> Scope4/1, NOR/1, D Flip-Flop1/1
  D Flip-Flop/2 -> Subsystem3/1(preset), Scope/2  "preset"
  Constant1/1 -> Cast To Boolean1/1
  Subsystem4/1(Q) -> B1/1, Scope6/1  "out"
  Subsystem3/1(Q) -> B3/1, Scope/1  "out"
  Delay1/1 -> Scope8/3, Subsystem6/2(clk)  "clk"
  Delay/1 -> Scope/3, Subsystem3/2(clk)  "clk"
  Subsystem5/1(Q) -> B0/1, Scope7/1  "out"
  D Flip-Flop5/2 -> Subsystem3/4(clear), Subsystem6/4(clear), Subsystem4/4(clear), Subsystem5/4(clear)
  D Flip-Flop5/1 -> Cast To Double/1, Scope9/1
  Cast To Double/1 -> SOC/1

== system SAR_ADC_Resistive_DAC_SinInput_HighSpeed_12072024/SAR/Subsystem3 ==
  preset : Inport
  clk : Inport  Port=2
  input : Inport  Port=3
  clear : Inport  Port=4
  NOT : Logic  Operator=NOT  IconShape=distinctive  AllPortsSameDT=off  OutDataTypeStr=boolean
  Subsystem : Subsystem
  Subsystem1 : Subsystem
  Q : Outport
  ~Q : Outport  Port=2
  wires:
  clk/1 -> Subsystem1/3(clock), NOT/1
  Subsystem/1(Q) -> Subsystem1/2(D)
  NOT/1 -> Subsystem/3(clock)
  preset/1 -> Subsystem1/1(preset), Subsystem/1(preset)
  clear/1 -> Subsystem/4(clear), Subsystem1/4(clear)
  input/1 -> Subsystem/2(D)
  Subsystem1/1(Q) -> Q/1  "output"
  Subsystem1/2(~Q) -> ~Q/1

== system SAR_ADC_Resistive_DAC_SinInput_HighSpeed_12072024/SAR/Subsystem4 ==
  preset : Inport
  clk : Inport  Port=2
  input : Inport  Port=3
  clear : Inport  Port=4
  NOT : Logic  Operator=NOT  IconShape=distinctive  AllPortsSameDT=off  OutDataTypeStr=boolean
  Subsystem : Subsystem
  Subsystem1 : Subsystem
  Q : Outport
  ~Q : Outport  Port=2
  wires:
  clk/1 -> Subsystem1/3(clock), NOT/1
  Subsystem/1(Q) -> Subsystem1/2(D)
  NOT/1 -> Subsystem/3(clock)
  preset/1 -> Subsystem1/1(preset), Subsystem/1(preset)
  clear/1 -> Subsystem/4(clear), Subsystem1/4(clear)
  input/1 -> Subsystem/2(D)
  Subsystem1/1(Q) -> Q/1  "output"
  Subsystem1/2(~Q) -> ~Q/1

== system SAR_ADC_Resistive_DAC_SinInput_HighSpeed_12072024/SAR/Subsystem5 ==
  preset : Inport
  clk : Inport  Port=2
  input : Inport  Port=3
  clear : Inport  Port=4
  NOT : Logic  Operator=NOT  IconShape=distinctive  AllPortsSameDT=off  OutDataTypeStr=boolean
  Subsystem : Subsystem
  Subsystem1 : Subsystem
  Q : Outport
  ~Q : Outport  Port=2
  wires:
  clk/1 -> Subsystem1/3(clock), NOT/1
  Subsystem/1(Q) -> Subsystem1/2(D)
  NOT/1 -> Subsystem/3(clock)
  preset/1 -> Subsystem1/1(preset), Subsystem/1(preset)
  clear/1 -> Subsystem/4(clear), Subsystem1/4(clear)
  input/1 -> Subsystem/2(D)
  Subsystem1/1(Q) -> Q/1  "output"
  Subsystem1/2(~Q) -> ~Q/1

== system SAR_ADC_Resistive_DAC_SinInput_HighSpeed_12072024/SAR/Subsystem6 ==
  preset : Inport
  clk : Inport  Port=2
  input : Inport  Port=3
  clear : Inport  Port=4
  NOT : Logic  Operator=NOT  IconShape=distinctive  AllPortsSameDT=off  OutDataTypeStr=boolean
  Subsystem : Subsystem
  Subsystem1 : Subsystem
  Q : Outport
  ~Q : Outport  Port=2
  wires:
  clk/1 -> Subsystem1/3(clock), NOT/1
  Subsystem/1(Q) -> Subsystem1/2(D)
  NOT/1 -> Subsystem/3(clock)
  preset/1 -> Subsystem1/1(preset), Subsystem/1(preset)
  clear/1 -> Subsystem/4(clear), Subsystem1/4(clear)
  input/1 -> Subsystem/2(D)
  Subsystem1/1(Q) -> Q/1  "output"
  Subsystem1/2(~Q) -> ~Q/1

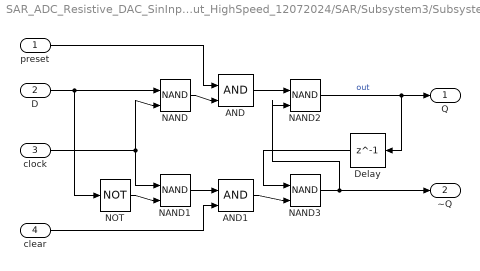
== system SAR_ADC_Resistive_DAC_SinInput_HighSpeed_12072024/SAR/Subsystem3/Subsystem ==
  preset : Inport
  D : Inport  Port=2
  clock : Inport  Port=3
  clear : Inport  Port=4
  AND : Logic  IconShape=distinctive  AllPortsSameDT=off  OutDataTypeStr=boolean
  AND1 : Logic  IconShape=distinctive  AllPortsSameDT=off  OutDataTypeStr=boolean
  Delay : Delay  DelayLength=1
  NAND{,1..3} (4 alike) : Logic  Operator=NAND  IconShape=distinctive  AllPortsSameDT=off  OutDataTypeStr=boolean
  NOT : Logic  Operator=NOT  IconShape=distinctive  AllPortsSameDT=off  OutDataTypeStr=boolean
  Q : Outport
  ~Q : Outport  Port=2
  wires:
  Delay/1 -> NAND3/1
  NOT/1 -> NAND1/2
  NAND1/1 -> AND1/1
  AND/1 -> NAND2/1
  NAND3/1 -> ~Q/1, NAND2/2
  D/1 -> NOT/1, NAND/1
  AND1/1 -> NAND3/2
  NAND/1 -> AND/2
  NAND2/1 -> Q/1, Delay/1  "out"
  clock/1 -> NAND/2, NAND1/1
  preset/1 -> AND/1
  clear/1 -> AND1/2

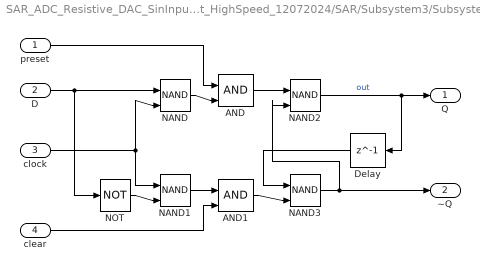
== system SAR_ADC_Resistive_DAC_SinInput_HighSpeed_12072024/SAR/Subsystem3/Subsystem1 ==
  preset : Inport
  D : Inport  Port=2
  clock : Inport  Port=3
  clear : Inport  Port=4
  AND : Logic  IconShape=distinctive  AllPortsSameDT=off  OutDataTypeStr=boolean
  AND1 : Logic  IconShape=distinctive  AllPortsSameDT=off  OutDataTypeStr=boolean
  Delay : Delay  DelayLength=1
  NAND{,1..3} (4 alike) : Logic  Operator=NAND  IconShape=distinctive  AllPortsSameDT=off  OutDataTypeStr=boolean
  NOT : Logic  Operator=NOT  IconShape=distinctive  AllPortsSameDT=off  OutDataTypeStr=boolean
  Q : Outport
  ~Q : Outport  Port=2
  wires:
  Delay/1 -> NAND3/1
  NOT/1 -> NAND1/2
  NAND1/1 -> AND1/1
  AND/1 -> NAND2/1
  NAND3/1 -> ~Q/1, NAND2/2
  D/1 -> NOT/1, NAND/1
  AND1/1 -> NAND3/2
  NAND/1 -> AND/2
  NAND2/1 -> Q/1, Delay/1  "out"
  clock/1 -> NAND/2, NAND1/1
  preset/1 -> AND/1
  clear/1 -> AND1/2

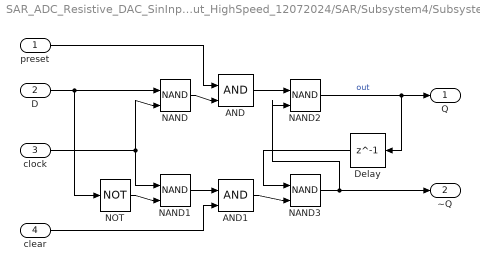
== system SAR_ADC_Resistive_DAC_SinInput_HighSpeed_12072024/SAR/Subsystem4/Subsystem ==
  preset : Inport
  D : Inport  Port=2
  clock : Inport  Port=3
  clear : Inport  Port=4
  AND : Logic  IconShape=distinctive  AllPortsSameDT=off  OutDataTypeStr=boolean
  AND1 : Logic  IconShape=distinctive  AllPortsSameDT=off  OutDataTypeStr=boolean
  Delay : Delay  DelayLength=1
  NAND{,1..3} (4 alike) : Logic  Operator=NAND  IconShape=distinctive  AllPortsSameDT=off  OutDataTypeStr=boolean
  NOT : Logic  Operator=NOT  IconShape=distinctive  AllPortsSameDT=off  OutDataTypeStr=boolean
  Q : Outport
  ~Q : Outport  Port=2
  wires:
  Delay/1 -> NAND3/1
  NOT/1 -> NAND1/2
  NAND1/1 -> AND1/1
  AND/1 -> NAND2/1
  NAND3/1 -> ~Q/1, NAND2/2
  D/1 -> NOT/1, NAND/1
  AND1/1 -> NAND3/2
  NAND/1 -> AND/2
  NAND2/1 -> Q/1, Delay/1  "out"
  clock/1 -> NAND/2, NAND1/1
  preset/1 -> AND/1
  clear/1 -> AND1/2

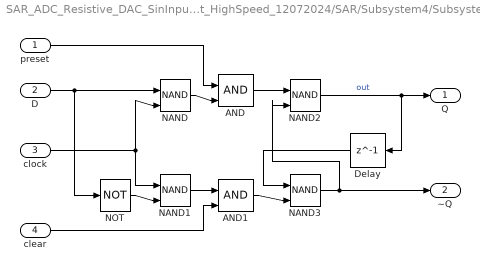
== system SAR_ADC_Resistive_DAC_SinInput_HighSpeed_12072024/SAR/Subsystem4/Subsystem1 ==
  preset : Inport
  D : Inport  Port=2
  clock : Inport  Port=3
  clear : Inport  Port=4
  AND : Logic  IconShape=distinctive  AllPortsSameDT=off  OutDataTypeStr=boolean
  AND1 : Logic  IconShape=distinctive  AllPortsSameDT=off  OutDataTypeStr=boolean
  Delay : Delay  DelayLength=1
  NAND{,1..3} (4 alike) : Logic  Operator=NAND  IconShape=distinctive  AllPortsSameDT=off  OutDataTypeStr=boolean
  NOT : Logic  Operator=NOT  IconShape=distinctive  AllPortsSameDT=off  OutDataTypeStr=boolean
  Q : Outport
  ~Q : Outport  Port=2
  wires:
  Delay/1 -> NAND3/1
  NOT/1 -> NAND1/2
  NAND1/1 -> AND1/1
  AND/1 -> NAND2/1
  NAND3/1 -> ~Q/1, NAND2/2
  D/1 -> NOT/1, NAND/1
  AND1/1 -> NAND3/2
  NAND/1 -> AND/2
  NAND2/1 -> Q/1, Delay/1  "out"
  clock/1 -> NAND/2, NAND1/1
  preset/1 -> AND/1
  clear/1 -> AND1/2

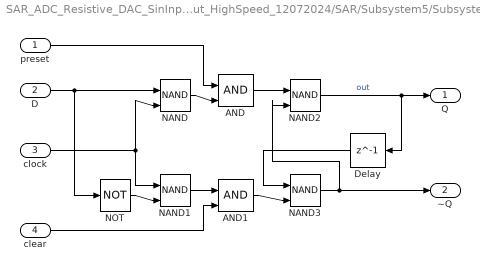
== system SAR_ADC_Resistive_DAC_SinInput_HighSpeed_12072024/SAR/Subsystem5/Subsystem ==
  preset : Inport
  D : Inport  Port=2
  clock : Inport  Port=3
  clear : Inport  Port=4
  AND : Logic  IconShape=distinctive  AllPortsSameDT=off  OutDataTypeStr=boolean
  AND1 : Logic  IconShape=distinctive  AllPortsSameDT=off  OutDataTypeStr=boolean
  Delay : Delay  DelayLength=1
  NAND{,1..3} (4 alike) : Logic  Operator=NAND  IconShape=distinctive  AllPortsSameDT=off  OutDataTypeStr=boolean
  NOT : Logic  Operator=NOT  IconShape=distinctive  AllPortsSameDT=off  OutDataTypeStr=boolean
  Q : Outport
  ~Q : Outport  Port=2
  wires:
  Delay/1 -> NAND3/1
  NOT/1 -> NAND1/2
  NAND1/1 -> AND1/1
  AND/1 -> NAND2/1
  NAND3/1 -> ~Q/1, NAND2/2
  D/1 -> NOT/1, NAND/1
  AND1/1 -> NAND3/2
  NAND/1 -> AND/2
  NAND2/1 -> Q/1, Delay/1  "out"
  clock/1 -> NAND/2, NAND1/1
  preset/1 -> AND/1
  clear/1 -> AND1/2

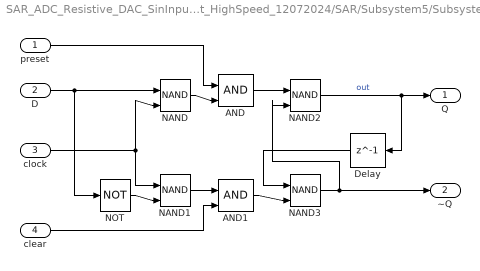
== system SAR_ADC_Resistive_DAC_SinInput_HighSpeed_12072024/SAR/Subsystem5/Subsystem1 ==
  preset : Inport
  D : Inport  Port=2
  clock : Inport  Port=3
  clear : Inport  Port=4
  AND : Logic  IconShape=distinctive  AllPortsSameDT=off  OutDataTypeStr=boolean
  AND1 : Logic  IconShape=distinctive  AllPortsSameDT=off  OutDataTypeStr=boolean
  Delay : Delay  DelayLength=1
  NAND{,1..3} (4 alike) : Logic  Operator=NAND  IconShape=distinctive  AllPortsSameDT=off  OutDataTypeStr=boolean
  NOT : Logic  Operator=NOT  IconShape=distinctive  AllPortsSameDT=off  OutDataTypeStr=boolean
  Q : Outport
  ~Q : Outport  Port=2
  wires:
  Delay/1 -> NAND3/1
  NOT/1 -> NAND1/2
  NAND1/1 -> AND1/1
  AND/1 -> NAND2/1
  NAND3/1 -> ~Q/1, NAND2/2
  D/1 -> NOT/1, NAND/1
  AND1/1 -> NAND3/2
  NAND/1 -> AND/2
  NAND2/1 -> Q/1, Delay/1  "out"
  clock/1 -> NAND/2, NAND1/1
  preset/1 -> AND/1
  clear/1 -> AND1/2

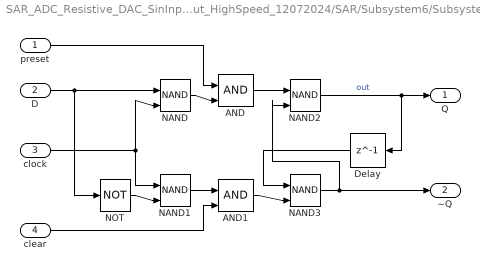
== system SAR_ADC_Resistive_DAC_SinInput_HighSpeed_12072024/SAR/Subsystem6/Subsystem ==
  preset : Inport
  D : Inport  Port=2
  clock : Inport  Port=3
  clear : Inport  Port=4
  AND : Logic  IconShape=distinctive  AllPortsSameDT=off  OutDataTypeStr=boolean
  AND1 : Logic  IconShape=distinctive  AllPortsSameDT=off  OutDataTypeStr=boolean
  Delay : Delay  DelayLength=1
  NAND{,1..3} (4 alike) : Logic  Operator=NAND  IconShape=distinctive  AllPortsSameDT=off  OutDataTypeStr=boolean
  NOT : Logic  Operator=NOT  IconShape=distinctive  AllPortsSameDT=off  OutDataTypeStr=boolean
  Q : Outport
  ~Q : Outport  Port=2
  wires:
  Delay/1 -> NAND3/1
  NOT/1 -> NAND1/2
  NAND1/1 -> AND1/1
  AND/1 -> NAND2/1
  NAND3/1 -> ~Q/1, NAND2/2
  D/1 -> NOT/1, NAND/1
  AND1/1 -> NAND3/2
  NAND/1 -> AND/2
  NAND2/1 -> Q/1, Delay/1  "out"
  clock/1 -> NAND/2, NAND1/1
  preset/1 -> AND/1
  clear/1 -> AND1/2

== system SAR_ADC_Resistive_DAC_SinInput_HighSpeed_12072024/SAR/Subsystem6/Subsystem1 ==
  preset : Inport
  D : Inport  Port=2
  clock : Inport  Port=3
  clear : Inport  Port=4
  AND : Logic  IconShape=distinctive  AllPortsSameDT=off  OutDataTypeStr=boolean
  AND1 : Logic  IconShape=distinctive  AllPortsSameDT=off  OutDataTypeStr=boolean
  Delay : Delay  DelayLength=1
  NAND{,1..3} (4 alike) : Logic  Operator=NAND  IconShape=distinctive  AllPortsSameDT=off  OutDataTypeStr=boolean
  NOT : Logic  Operator=NOT  IconShape=distinctive  AllPortsSameDT=off  OutDataTypeStr=boolean
  Q : Outport
  ~Q : Outport  Port=2
  wires:
  Delay/1 -> NAND3/1
  NOT/1 -> NAND1/2
  NAND1/1 -> AND1/1
  AND/1 -> NAND2/1
  NAND3/1 -> ~Q/1, NAND2/2
  D/1 -> NOT/1, NAND/1
  AND1/1 -> NAND3/2
  NAND/1 -> AND/2
  NAND2/1 -> Q/1, Delay/1  "out"
  clock/1 -> NAND/2, NAND1/1
  preset/1 -> AND/1
  clear/1 -> AND1/2
